simulink model "HouseThermalWithInputData"  (R2019a)
settings: Solver=FixedStepAuto  StartTime=0.0  StopTime=24*60*60  FixedStep=Ts  MaxStep=50  RelTol=1e-3  AbsTol=1e-3  EnableMultiTasking=on
PreLoadFcn:
  | %Load Input Data
  | % prepareInputData
  | load('HouseThermalTestData');
  | 
  | % Time step and initial conditions
  | PIDFault = false;
  | BlockageOn = false;
  | Ts = 5;
  | load InitialConditions.mat
  | 
  | % Walls
  | lenHouse   = 30;          % House length [m]
  | widHouse   = 10;          % House width [m]
  | htHouse     = 4;            % House height [m]
  | LWall           = 0.2;         % Wall thickness [m]
  | wallDensity = 1920;      % Density [kg/m^3]
  | c_wall          = 835;        % Specific heat [J/kg/K]
  | kWall            = 0.038;    % Thermal conductivity [W/m/K]
  | 
  | % Windows
  | n1_window       = 3;          % Number or windows in room 1
  | n2_window       = 2;          % Number or windows in room 2
  | n3_window       = 2;          % Number or windows in room 3
  | n4_window       = 2;          % Number or windows in room 4
  | htWindows       = 1;          % Height of windows [m]
  | widWindows      = 1;          % Width of windows  [m]
  | LWindow           = 0.01;     % Thickenss of windows [m]
  | windowDensity = 2700;    % Density [kg/m^3]
  | c_window          = 840;      % Specific heat [J/kg/K]
  | kWindow           = 0.78;     % Thermal conductivity [W/m/K]
  | 
  | 
  | % Roof
  | pitRoof         = 40/180/pi;   % Roof pitch (40 deg)
  | LRoof           = 0.2;             % Roof thickness [m]
  | roofDensity = 32;              % Roof density (Glass fiber) [kg/m^3]
  | c_roof          = 835;            % Specific heat [J/kg/K]
  | kRoof           = 0.038;         % Thermal conductivity [W/m/K]
  | 
  | % Radiators
  | %% Exchange area with air
  | S_radiator1 = 5;     % [m^2]
  | S_radiator2 = 5;     % [m^2]
  | S_radiator3 = 5;     % [m^2]
  | S_radiator4 = 5;     % [m^2]
  | %% Convective heat transfer coefficient radiator -> room
  | h_radiator1 = 100;  %  [W/(m^2 * K)]
  | h_radiator2 = 100;  %  [W/(m^2 * K)]
  | h_radiator3 = 100;  %  [W/(m^2 * K)]
  | h_radiator4 = 100;  %  [W/(m^2 * K)]
  | 
  | % Convective heat transfer coefficients [W/M^2/K]
  | h_air_wall         = 18;    % Indoor air->walls
  | h_wall_atm       = 20;   % Walls -> atmosphere
  | h_air_window    = 16;   % Indoor air -> windows
  | h_window_atm = 18;    % Windows -> atmosphere
  | h_air_roof         = 8;   % Indoor air -> roof
  | h_roof_atm      = 20;    % Roof -> atmosphere
  | 
  | %Air
  | ... (+37 lines)
libraries: fl_lib x116, nesl_utility x15, SimscapeFluids_lib x8, simulink x1
(part 4 of 4)

== system HouseThermalWithInputData/House thermal network/Variant Subsystem/Blockage ==
  Local Restriction (TL) : fl_lib/Thermal Liquid/Elements/Local Restriction (TL)  restriction_area=5e-3 m^2  area=0.01 m^2  length=0.1 m  Cd=0.7  pressure_recovery=1  Re_c=12  mdot_A_specify=off  mdot_A_priority=None  mdot_A=1 kg/s  mdot_A_nominal_specify=off  mdot_A_nominal_unit=kg/s  mdot_A_nominal_value=1
      settings: SourceProductName=Simscape  SourceProductBaseCode=SS
  A : PMIOPort  Side=Left
  B : PMIOPort  Port=2  Side=Right
  connections:
  Local Restriction (TL)/LConn1 -- A/RConn1
  Local Restriction (TL)/RConn1 -- B/RConn1

== system HouseThermalWithInputData/House thermal network/Variant Subsystem/Normal ==
  A : PMIOPort  Side=Left
  B : PMIOPort  Port=2  Side=Right
  connections:
  A/RConn1 -- B/RConn1
